simulink model "Filtration"  (R2022b)
settings: Solver=VariableStepAuto  StartTime=0.0  StopTime=30  RelTol=1e-3
libraries: dsparch4 x6, dspstat3 x2
settings Model: Creator=admin  LastModifiedBy=anver
settings DebuggingCC: UnconnectedInputMsg=warning  UnconnectedOutputMsg=warning  UnconnectedLineMsg=warning
settings ModelReferenceCC: EnableRefExpFcnMdlSchedulingChecks=on
settings RTWCC: DLArmComputeVersion=19.05

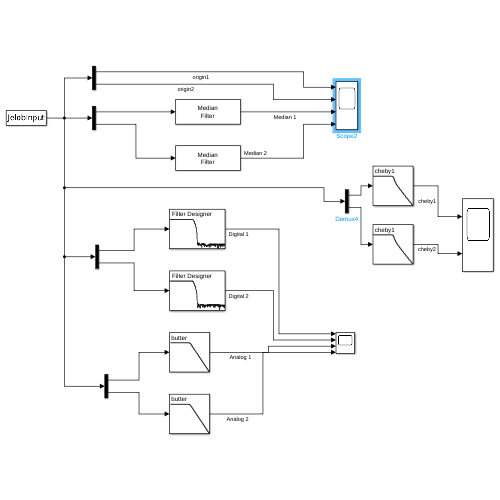
[thumbnail: Simulink's stored preview of the top-level diagram]
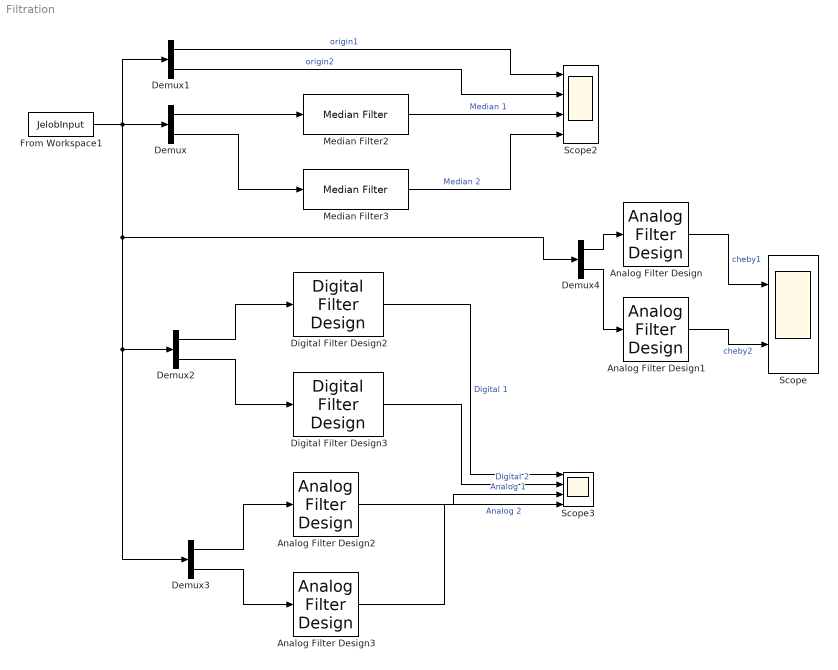
== system Filtration ==
  Analog Filter Design : dsparch4/Analog Filter Design  method=Chebyshev I  filttype=Lowpass  N=8  Wlo=30  Whi=80  Rp=2  Rs=40
  Analog Filter Design1 : dsparch4/Analog Filter Design  method=Chebyshev I  filttype=Lowpass  N=8  Wlo=30  Whi=80  Rp=2  Rs=40
  Analog Filter Design2 : dsparch4/Analog Filter Design  method=Butterworth  filttype=Lowpass  N=8  Wlo=30  Whi=80  Rp=2  Rs=40
  Analog Filter Design3 : dsparch4/Analog Filter Design  method=Butterworth  filttype=Lowpass  N=8  Wlo=30  Whi=80  Rp=2  Rs=40
  Demux{,1..4} (5 alike) : Demux  Outputs=2
  Digital Filter Design2 : dsparch4/Digital Filter Design  mwdsp_browser_bugfix_var=off
  Digital Filter Design3 : dsparch4/Digital Filter Design  mwdsp_browser_bugfix_var=off
  From Workspace1 : FromWorkspace  VariableName=JelobInput
  Median Filter2 : dspstat3/Median Filter  WindowLength=1000  SimulateUsing=Interpreted execution
  Median Filter3 : dspstat3/Median Filter  WindowLength=1000  SimulateUsing=Interpreted execution
  Scope : Scope  NumInputPorts=2
  Scope2 : Scope  NumInputPorts=4
  Scope3 : Scope  NumInputPorts=4
  wires:
  From Workspace1/1 -> Demux4/1, Demux3/1, Demux2/1, Demux1/1, Demux/1
  Median Filter2/1 -> Scope2/3  "Median 1"
  Median Filter3/1 -> Scope2/4  "Median 2"
  Demux/1 -> Median Filter2/1
  Demux/2 -> Median Filter3/1
  Demux1/2 -> Scope2/2  "origin2"
  Demux1/1 -> Scope2/1  "origin1"
  Demux2/1 -> Digital Filter Design2/1
  Demux2/2 -> Digital Filter Design3/1
  Digital Filter Design2/1 -> Scope3/1  "Digital 1"
  Digital Filter Design3/1 -> Scope3/2  "Digital 2"
  Demux3/1 -> Analog Filter Design2/1
  Demux3/2 -> Analog Filter Design3/1
  Analog Filter Design2/1 -> Scope3/3  "Analog 1"
  Analog Filter Design3/1 -> Scope3/4  "Analog 2"
  Demux4/2 -> Analog Filter Design1/1
  Demux4/1 -> Analog Filter Design/1
  Analog Filter Design/1 -> Scope/1  "cheby1"
  Analog Filter Design1/1 -> Scope/2  "cheby2"
